simulink library "AeroLib"  (Simulink 6.0)
settings: Solver=ode45  SolverMode=SingleTasking  StartTime=0.0  StopTime=10.0  RelTol=1e-3
undefined symbols (not defined in the file): Aero, Ap, Atm, Control, Controls, Eng, Flight_cg, Flight_DamperON, Flight_delta_isa, Flight_DeltaSpiral, Flight_InertiaSelect, Flight_ixx, Flight_ixz, Flight_iyy, Flight_izz, Flight_latitude, Flight_LoiterLenght, Flight_LoiterMode, Flight_LoiterRadius, Flight_longitude, Flight_MaxTargetPoints, Flight_SensorsON, Flight_TimeStep, Flight_TowerWind_X, Flight_TowerWind_Y, Flight_TowerWind_Z, Flight_TowerWindON, Flight_Trimming, Flight_TurbON, Flight_weight, Flight_WindGustON, Flight_WindShearON, Flight_ycg, Flight_zcg, Geom, Lgear, Mass, PEG_CDwbnp, PEG_CLht, PEG_CLht_elev, PEG_CLwbnp, PEG_CMht, PEG_CMwbnp, PEG_CNbeta, PEG_CNr, PEG_CNrud, PEG_CRail, PEG_CRbeta, PEG_CRp, PEG_CRrud, PEG_CYbeta, PEG_CYrud, pow, Sensors
libraries: AeroLib x133, simulink3 x49, simulink x37, aerospace x11
(part 6 of 7)

== system AeroLib/AtmosphericData/FAA_Std_Gust/Turbulence U/Filter_U2 ==
  Noise : Inport  Port=1  LatchInput=off
  Freq : Inport  Port=2  LatchInput=off
  From_Reset : Inport  Port=3  LatchInput=off
  Constant : Constant  Value=0
  Stateless_Integrator : AeroLib/AMS_StatelessFilters/Stateless_Integrator
  Sum : Sum  Inputs=|+-  SaturateOnIntegerOverflow=on  InputSameDT=on
  err_freq : Product  SaturateOnIntegerOverflow=on  InputSameDT=on
  FiltNoise : Outport
  wires:
  From_Reset/1 -> Stateless_Integrator/1
  Constant/1 -> Stateless_Integrator/2
  err_freq/1 -> Stateless_Integrator/3
  Freq/1 -> err_freq/1
  Sum/1 -> err_freq/2  "err"
  Noise/1 -> Sum/1  "noise_u"
  Stateless_Integrator/1 -> FiltNoise/1, Sum/2

== system AeroLib/AtmosphericData/FAA_Std_Gust/Turbulence V/Filter_V1 ==
  Noise : Inport  Port=1  LatchInput=off
  Freq : Inport  Port=2  LatchInput=off
  From_Reset : Inport  Port=3  LatchInput=off
  Constant : Constant  Value=0
  Stateless_Integrator : AeroLib/AMS_StatelessFilters/Stateless_Integrator
  Sum : Sum  Inputs=|+-  SaturateOnIntegerOverflow=on  InputSameDT=on
  err_freq : Product  SaturateOnIntegerOverflow=on  InputSameDT=on
  FiltNoise : Outport
  wires:
  Stateless_Integrator/1 -> Sum/2, FiltNoise/1
  Noise/1 -> Sum/1  "noise_u"
  Sum/1 -> err_freq/2  "err"
  Freq/1 -> err_freq/1
  err_freq/1 -> Stateless_Integrator/3
  Constant/1 -> Stateless_Integrator/2
  From_Reset/1 -> Stateless_Integrator/1

== system AeroLib/AtmosphericData/FAA_Std_Gust/Turbulence V/Filter_V2 ==
  Noise : Inport  Port=1  LatchInput=off
  Freq : Inport  Port=2  LatchInput=off
  From_Reset : Inport  Port=3  LatchInput=off
  Constant : Constant  Value=0
  Stateless_Integrator : AeroLib/AMS_StatelessFilters/Stateless_Integrator
  Sum : Sum  Inputs=|+-  SaturateOnIntegerOverflow=on  InputSameDT=on
  err_freq : Product  SaturateOnIntegerOverflow=on  InputSameDT=on
  FiltNoise : Outport
  wires:
  From_Reset/1 -> Stateless_Integrator/1
  Constant/1 -> Stateless_Integrator/2
  err_freq/1 -> Stateless_Integrator/3
  Freq/1 -> err_freq/1
  Sum/1 -> err_freq/2  "err"
  Noise/1 -> Sum/1  "noise_u"
  Stateless_Integrator/1 -> FiltNoise/1, Sum/2

== system AeroLib/AtmosphericData/FAA_Std_Gust/Turbulence V/Filter_V3 ==
  Noise : Inport  Port=1  LatchInput=off
  Freq : Inport  Port=2  LatchInput=off
  From_Reset : Inport  Port=3  LatchInput=off
  Constant : Constant  Value=0
  Stateless_Integrator : AeroLib/AMS_StatelessFilters/Stateless_Integrator
  Sum : Sum  Inputs=|+-  SaturateOnIntegerOverflow=on  InputSameDT=on
  err_freq : Product  SaturateOnIntegerOverflow=on  InputSameDT=on
  FiltNoise : Outport
  wires:
  Stateless_Integrator/1 -> Sum/2, FiltNoise/1
  Noise/1 -> Sum/1  "noise_u"
  Sum/1 -> err_freq/2  "err"
  Freq/1 -> err_freq/1
  err_freq/1 -> Stateless_Integrator/3
  Constant/1 -> Stateless_Integrator/2
  From_Reset/1 -> Stateless_Integrator/1

== system AeroLib/AtmosphericData/FAA_Std_Gust/Turbulence W/Filter_W1 ==
  Noise : Inport  Port=1  LatchInput=off
  Freq : Inport  Port=2  LatchInput=off
  From_Reset : Inport  Port=3  LatchInput=off
  Constant : Constant  Value=0
  Stateless_Integrator : AeroLib/AMS_StatelessFilters/Stateless_Integrator
  Sum : Sum  Inputs=|+-  SaturateOnIntegerOverflow=on  InputSameDT=on
  err_freq : Product  SaturateOnIntegerOverflow=on  InputSameDT=on
  FiltNoise : Outport
  wires:
  Stateless_Integrator/1 -> Sum/2, FiltNoise/1
  Noise/1 -> Sum/1  "noise_u"
  Sum/1 -> err_freq/2  "err"
  Freq/1 -> err_freq/1
  err_freq/1 -> Stateless_Integrator/3
  Constant/1 -> Stateless_Integrator/2
  From_Reset/1 -> Stateless_Integrator/1

== system AeroLib/AtmosphericData/FAA_Std_Gust/Turbulence W/Filter_W2 ==
  Noise : Inport  Port=1  LatchInput=off
  Freq : Inport  Port=2  LatchInput=off
  From_Reset : Inport  Port=3  LatchInput=off
  Constant : Constant  Value=0
  Stateless_Integrator : AeroLib/AMS_StatelessFilters/Stateless_Integrator
  Sum : Sum  Inputs=|+-  SaturateOnIntegerOverflow=on  InputSameDT=on
  err_freq : Product  SaturateOnIntegerOverflow=on  InputSameDT=on
  FiltNoise : Outport
  wires:
  From_Reset/1 -> Stateless_Integrator/1
  Constant/1 -> Stateless_Integrator/2
  err_freq/1 -> Stateless_Integrator/3
  Freq/1 -> err_freq/1
  Sum/1 -> err_freq/2  "err"
  Noise/1 -> Sum/1  "noise_u"
  Stateless_Integrator/1 -> FiltNoise/1, Sum/2

== system AeroLib/AtmosphericData/FAA_Std_Gust/Turbulence W/Filter_W3 ==
  Noise : Inport  Port=1  LatchInput=off
  Freq : Inport  Port=2  LatchInput=off
  From_Reset : Inport  Port=3  LatchInput=off
  Constant : Constant  Value=0
  Stateless_Integrator : AeroLib/AMS_StatelessFilters/Stateless_Integrator
  Sum : Sum  Inputs=|+-  SaturateOnIntegerOverflow=on  InputSameDT=on
  err_freq : Product  SaturateOnIntegerOverflow=on  InputSameDT=on
  FiltNoise : Outport
  wires:
  Stateless_Integrator/1 -> Sum/2, FiltNoise/1
  Noise/1 -> Sum/1  "noise_u"
  Sum/1 -> err_freq/2  "err"
  Freq/1 -> err_freq/1
  err_freq/1 -> Stateless_Integrator/3
  Constant/1 -> Stateless_Integrator/2
  From_Reset/1 -> Stateless_Integrator/1

== system AeroLib/Autopilot/Autopilot/Dampers/Pitch_Damper ==
  From_Reset : Inport  Port=1  LatchInput=off
  From_INS : Inport  Port=2  LatchInput=off
  Alpha : Inport  Port=3  LatchInput=off
  From_Prop : Inport  Port=4  LatchInput=off
  From_Inputs : Inport  Port=5  LatchInput=off
  Limit_Alpha_and_Speed : Subsystem
  Pitch_damp : Subsystem  mask{Kq=Ap.Alt.damph, Kd=Ap.Alt.dgain}
      mask prompts: Kq "Damphing"; Kd "Derivative"
  Sum : Sum  Inputs=|++  SaturateOnIntegerOverflow=on  InputSameDT=on
  Elev_cmd : Outport
  wires:
  From_Reset/1 -> Limit_Alpha_and_Speed/2(Reset)
  From_INS/1 -> Limit_Alpha_and_Speed/1(TAS), Pitch_damp/1(From_INS)
  Limit_Alpha_and_Speed/1(Elev_minSpeed) -> Sum/2
  Pitch_damp/1(Elev_cmd) -> Sum/1
  Alpha/1 -> Limit_Alpha_and_Speed/4(Alpha)
  From_Prop/1 -> Limit_Alpha_and_Speed/3(From_Prop)
  Sum/1 -> Elev_cmd/1
  From_Inputs/1 -> Limit_Alpha_and_Speed/5(From_Inputs)

== system AeroLib/Autopilot/Autopilot/Dampers/Roll_Damper ==
  From_Sen : Inport  Port=1  LatchInput=off
  From_Reset : Inport  Port=2  LatchInput=off
  Phi Limit : Subsystem
  Roll_damp : Subsystem  mask{Kp=Ap.Track.damph, Kd=Ap.Track.dgain}
      mask prompts: Kp "Damphing"; Kd "Derivative"
  Sum1 : Sum  Inputs=|++  SaturateOnIntegerOverflow=on  InputSameDT=on
  Ail_cmd : Outport
  wires:
  From_Reset/1 -> Roll_damp/2(Reset_In), Phi Limit/1(Reset_In)
  From_Sen/1 -> Phi Limit/2(Phi), Roll_damp/1(From_Sen)
  Roll_damp/1(Ail_cmd) -> Sum1/1
  Sum1/1 -> Ail_cmd/1
  Phi Limit/1(Ail) -> Sum1/2

== system AeroLib/Autopilot/Autopilot/Dampers/Yaw_Damper ==
  Ny : Inport  Port=1  LatchInput=off
  From_Reset : Inport  Port=2  LatchInput=off
  Gain : Gain  Gain=Ap.Ny.gain  SaturateOnIntegerOverflow=on
  PID_Ny : Subsystem  mask(PID(2) Controller){P=Ap.Ny.pgain, I=Ap.Ny.igain, D=Ap.Ny.dgain}
      mask prompts: P "Proportional:"; I "Integral:"; D "Derivative:"
      mask help:
      | Enter Proportional(P), Integral(I), and Derivative(D) and divisor (N) terms.
      | P+I/s+Ds/(1/Ns+1)
      mask Help: This block implements a PID controller where parameters are entered for the Proportional, Integral and Derivative and divisor terms. Unmask this block to see how it works. The derivative term is implemented using an s/(s/N +1)  transfer function block. Making N large can create a "stiff" system.
      mask Display: disp('PID')
  Rud_cmd : Outport
  wires:
  From_Reset/1 -> PID_Ny/2(From_Reset)
  PID_Ny/1(Cmd) -> Rud_cmd/1
  Ny/1 -> Gain/1
  Gain/1 -> PID_Ny/1(Err)

== system AeroLib/Autopilot/Autopilot/Guidance/Loiter_modes ==
  note: Flight_LoiterMode
      | 1 - Spiral or circle
      | 2 - Serpentine
      | 3 - Lazy eight
  Target_N : Inport  Port=1  LatchInput=off
  From_FSC : Inport  Port=2  LatchInput=off
  From_Reset : Inport  Port=3  LatchInput=off
  Constant : Constant  Value=2
  Constant1 : Constant  Value=Flight_LoiterMode
  Demux : Demux  Outputs=2
  Last_point_data : Subsystem
  MinMax : MinMax  Inputs=2  SaturateOnIntegerOverflow=on  InputSameDT=on
  Multiport Switch : MultiPortSwitch  Inputs=2  SaturateOnIntegerOverflow=on  InputSameDT=on
  Mux : Mux  Inputs=2
  Mux1 : Mux  Inputs=2
  Serpentine_Loiter_mode : Subsystem
  Spiral_and_circle_Loiter_mode : Subsystem  TreatAsAtomicUnit=on
  Subsystem : Subsystem
  Track_Err : Outport
  Point_N : Outport  Port=2
  wires:
  Multiport Switch/1 -> Demux/1
  From_Reset/1 -> Spiral_and_circle_Loiter_mode/3(From_Reset), Serpentine_Loiter_mode/5(From_Reset)
  Mux/1 -> Multiport Switch/2
  Mux1/1 -> Multiport Switch/3
  MinMax/1 -> Multiport Switch/1
  Constant1/1 -> MinMax/1
  Constant/1 -> MinMax/2
  Demux/2 -> Point_N/1
  Demux/1 -> Track_Err/1
  Serpentine_Loiter_mode/2(Point_N) -> Mux1/2
  Serpentine_Loiter_mode/1(Track_Err) -> Mux1/1
  Spiral_and_circle_Loiter_mode/2(Point_N) -> Mux/2
  Spiral_and_circle_Loiter_mode/1(Track_Err) -> Mux/1
  Subsystem/1(Enable_com) -> Spiral_and_circle_Loiter_mode/Enable
  Last_point_data/3(LastTrack_rad) -> Spiral_and_circle_Loiter_mode/1(LastTrack), Serpentine_Loiter_mode/4(Track_last)
  Last_point_data/2(LastY_m) -> Serpentine_Loiter_mode/3(Y_last)
  Last_point_data/1(LastX_m) -> Serpentine_Loiter_mode/2(X_last)
  From_FSC/1 -> Serpentine_Loiter_mode/1(From_FSC), Last_point_data/1(From_Sensors), Spiral_and_circle_Loiter_mode/2(From_FSC)
  Target_N/1 -> Last_point_data/2(Target_N), Subsystem/1(Target_N)

== system AeroLib/Autopilot/Autopilot/Guidance/Target_Errors ==
  Y_req : Inport  Port=1  LatchInput=off
  X_Req : Inport  Port=2  LatchInput=off
  Speed_Req : Inport  Port=3  LatchInput=off
  Alt_Req : Inport  Port=4  LatchInput=off
  From_Prop : Inport  Port=5  LatchInput=off
  From_Inputs : Inport  Port=6  LatchInput=off
  From_Sen : Inport  Port=7  LatchInput=off
  AP_RATO : Subsystem
  Bus Selector3 : BusSelector  DialogController=Simulink.DDGSource_Bus  OutputSignals=IRU_RadarAlt_ft
  Constant : Constant  Value=0
  Switch : Switch  Threshold=0.5  SaturateOnIntegerOverflow=on  InputSameDT=on
  Switch1 : Switch  Threshold=0.5  SaturateOnIntegerOverflow=on  InputSameDT=on
  Target_Errors : AeroLib/Autopilot/Target_Errors
  ft--->m1 : Gain  Gain=1.01  SaturateOnIntegerOverflow=on
  Distance : Outport
  Speed_Err : Outport  Port=2
  Alt_Err : Outport  Port=3
  Bearing : Outport  Port=4
  Time_to_Go : Outport  Port=5
  Track_Err : Outport  Port=6
  wires:
  From_Sen/1 -> AP_RATO/1(FromSensor), Bus Selector3/1, Target_Errors/4
  Bus Selector3/1 -> ft--->m1/1  "<IRU_RadarAlt_ft>"
  AP_RATO/1(HoldAlt_ON) -> Switch1/2, Switch/2
  Target_Errors/6 -> Alt_Err/1
  Target_Errors/5 -> Bearing/1
  Target_Errors/4 -> Speed_Err/1
  Speed_Req/1 -> Target_Errors/3
  X_Req/1 -> Target_Errors/2
  Target_Errors/2 -> Time_to_Go/1
  Target_Errors/1 -> Distance/1
  Y_req/1 -> Target_Errors/1
  Target_Errors/3 -> Switch1/1
  From_Prop/1 -> AP_RATO/2(From_Prop)
  Switch/1 -> Target_Errors/5
  Alt_Req/1 -> Switch/1
  ft--->m1/1 -> Switch/3
  From_Inputs/1 -> AP_RATO/3(From_Inputs)
  Switch1/1 -> Track_Err/1
  Constant/1 -> Switch1/3

== system AeroLib/Autopilot/Autopilot/Guidance/Target_Selector ==
  Distance : Inport  Port=1  LatchInput=off
  PointsXY : Inport  Port=2  LatchInput=off
  PointsLatLon : Inport  Port=3  LatchInput=off
  From_Reset : Inport  Port=4  LatchInput=off
  Counter_Point : AeroLib/Autopilot/Counter_Point  MinDist=Ap.Target.MinDist
  Demux : Demux
  Demux1 : Demux  Outputs=2
  Fcn4 : Fcn  Expr=u+1
  Mem1 : Memory  X0=1000000000
  Saturation : Saturate  UpperLimit=Flight_MaxTargetPoints  LowerLimit=0
  Selector : Selector  InputType=Matrix  Elements=[2 ]  RowSrc=External  Rows=5  Columns=-1  InputPortWidth=4
  Selector1 : Selector  InputType=Matrix  Elements=[2 ]  RowSrc=External  Rows=5  Columns=-1  InputPortWidth=4
  Y_target : Outport
  X_target : Outport  Port=2
  V_req : Outport  Port=3
  Z_target : Outport  Port=4
  Point_N : Outport  Port=5
  Lat_target : Outport  Port=6
  Lon_target : Outport  Port=7
  wires:
  Saturation/1 -> Selector/2, Selector1/2
  Distance/1 -> Mem1/1
  Selector/1 -> Demux/1
  Fcn4/1 -> Saturation/1, Point_N/1
  Demux/1 -> X_target/1
  Demux/2 -> Y_target/1
  Demux/3 -> Z_target/1
  Demux/4 -> V_req/1
  PointsXY/1 -> Selector/1
  Counter_Point/1 -> Fcn4/1
  Mem1/1 -> Counter_Point/1
  From_Reset/1 -> Counter_Point/2
  Selector1/1 -> Demux1/1
  PointsLatLon/1 -> Selector1/1
  Demux1/1 -> Lat_target/1
  Demux1/2 -> Lon_target/1

== system AeroLib/Autopilot/GeodCoor to XY/Geo2orto/Geod_coor ==
  Lat_Init : Inport  Port=1  LatchInput=off
  Lat_Targ : Inport  Port=2  LatchInput=off
  DeltaLon : Inport  Port=3  LatchInput=off
  Product{,1..5} (6 alike) : Product  SaturateOnIntegerOverflow=on  InputSameDT=on
  Sum : Sum  Inputs=|++  SaturateOnIntegerOverflow=on  InputSameDT=on
  Sum1 : Sum  Inputs=|+-  SaturateOnIntegerOverflow=on  InputSameDT=on
  Trigonometric Function1 : Trigonometry
  Trigonometric Function2 : Trigonometry  Operator=cos
  Trigonometric Function3 : Trigonometry  Operator=cos
  Trigonometric Function4 : Trigonometry
  Trigonometric Function5 : Trigonometry
  Trigonometric Function6 : Trigonometry  Operator=cos
  P : Outport
  U : Outport  Port=2
  Q : Outport  Port=3
  wires:
  Trigonometric Function4/1 -> Product3/1, Product5/1
  Trigonometric Function6/1 -> Product2/2, Product4/2
  Lat_Init/1 -> Trigonometric Function4/1, Trigonometric Function6/1
  Trigonometric Function5/1 -> Product3/2, Product2/1
  Lat_Targ/1 -> Trigonometric Function3/1, Trigonometric Function5/1
  Trigonometric Function3/1 -> Product/1, Product1/1
  Trigonometric Function1/1 -> Product/2
  DeltaLon/1 -> Trigonometric Function1/1, Trigonometric Function2/1
  Trigonometric Function2/1 -> Product1/2
  Product/1 -> P/1
  Product3/1 -> Sum/1
  Product1/1 -> Product4/1, Product5/2
  Product4/1 -> Sum/2
  Sum/1 -> U/1
  Product2/1 -> Sum1/1
  Product5/1 -> Sum1/2
  Sum1/1 -> Q/1

== system AeroLib/EquationsOfMotion/Equations_of_Motion/EQM Six-DOF/EQM Forces ==
  Fext : Inport  Port=1  LatchInput=off
  Weight : Inport  Port=2  LatchInput=off
  Rate : Inport  Port=3  LatchInput=off
  Vb : Inport  Port=4  LatchInput=off
  Force_Vb_w : aerospace/Axes Transformations/3x3 cross product
  Gravity : Constant  Value=Atm.grav
  Product : Product  Inputs=*/  SaturateOnIntegerOverflow=on  InputSameDT=on
  Product1 : Product  Inputs=*/  SaturateOnIntegerOverflow=on  InputSameDT=on
  sum : Sum  SaturateOnIntegerOverflow=on  InputSameDT=on
  Accel : Outport
  wires:
  sum/1 -> Accel/1
  Product/1 -> sum/1
  Force_Vb_w/1 -> sum/2
  Fext/1 -> Product/1
  Vb/1 -> Force_Vb_w/1
  Rate/1 -> Force_Vb_w/2
  Weight/1 -> Product1/1
  Gravity/1 -> Product1/2
  Product1/1 -> Product/2

== system AeroLib/EquationsOfMotion/Equations_of_Motion/EQM Six-DOF/EQM Moments ==
  Moments : Inport  Port=1  LatchInput=off
  Inertia : Inport  Port=2  LatchInput=off
  Rates : Inport  Port=3  LatchInput=off
  Moment_Rates_Inertia : aerospace/Axes Transformations/3x3 cross product
  Product : Product  Inputs=/*  Multiplication=Matrix(*)  SaturateOnIntegerOverflow=on  InputSameDT=on
  matr_mult : Product  Multiplication=Matrix(*)  SaturateOnIntegerOverflow=on  InputSameDT=on
  sum1 : Sum  Inputs=+-  SaturateOnIntegerOverflow=on  InputSameDT=on
  pdot qdot rdot : Outport
  wires:
  Product/1 -> pdot qdot rdot/1
  Moment_Rates_Inertia/1 -> sum1/2
  matr_mult/1 -> Moment_Rates_Inertia/2
  Moments/1 -> sum1/1
  Rates/1 -> Moment_Rates_Inertia/1, matr_mult/2
  Inertia/1 -> matr_mult/1, Product/1
  sum1/1 -> Product/2

== system AeroLib/EquationsOfMotion/Equations_of_Motion/EQM Six-DOF/Geodetic_Frame_EQM ==
  note: LongitudeDot
      |
      |
      | LatitudeDot
  note: XYZ - Earth axis system
      |
      | X - pointing North
      | Y - pointing East
      | Z - pointing Down towards the center of the Earth
  VN : Inport  Port=1  LatchInput=off
  VE : Inport  Port=2  LatchInput=off
  Alt_m : Inport  Port=3  LatchInput=off
  Reset : Inport  Port=4  LatchInput=off
  Constant : Constant  Value=0
  Constant1 : Constant  Value=Flight_latitude
  Constant23 : Constant  Value=Flight_longitude
  Deg-->Rad : Gain  Gain=pi/180  SaturateOnIntegerOverflow=on
  Demux : Demux  Outputs=2
  Fcn5 : Fcn  Expr=u(2)*sin(u(1))
  LatitudeDot : Product  Inputs=/*  SaturateOnIntegerOverflow=on  InputSameDT=on
  LongitudeDot : Product  Inputs=*//  SaturateOnIntegerOverflow=on  InputSameDT=on
  Longitude_Bound : Subsystem
  Mux{,1..2,4} (4 alike) : Mux  Inputs=2
  Stateless_Integrator : AeroLib/AMS_StatelessFilters/Stateless_Integrator
  Stateless_Integrator1 : AeroLib/AMS_StatelessFilters/Stateless_Integrator
  Trigonometric Function : Trigonometry  Operator=cos
  WGS 84 : Subsystem
  Zero-->Eps : Subsystem
  latitude_Bound : Lookup  DialogController=Simulink.DDGSource  InputValues=[-2*pi -3*pi/2 -pi -pi/2 0 pi/2 pi 3*pi/2 2*pi]  OutputValues=[0 pi/2 0 -pi/2 0 pi/2 0 -pi/2 0]  SaturateOnIntegerOverflow=on
  rad-->deg : Gain  Gain=180/pi  SaturateOnIntegerOverflow=on
  Wander angle_rad : Outport
  Latitude_deg : Outport  Port=2
  Longitude_deg : Outport  Port=3
  GeodHeight_m : Outport  Port=4
  wires:
  Alt_m/1 -> WGS 84/2(Altitude_m)
  VN/1 -> LatitudeDot/2
  WGS 84/3(RadOfCurv_mer_m) -> LatitudeDot/1
  Longitude_Bound/2(Lat_deg) -> Latitude_deg/1
  Mux1/1 -> rad-->deg/1
  LongitudeDot/1 -> Mux4/2, Mux/1
  Mux/1 -> Stateless_Integrator1/3
  LatitudeDot/1 -> Mux/2
  Stateless_Integrator1/1 -> Demux/1
  Trigonometric Function/1 -> Zero-->Eps/1(In1)
  WGS 84/2(GeogHight_m) -> GeodHeight_m/1
  Zero-->Eps/1(Out1) -> LongitudeDot/2
  WGS 84/1(RadOfCurv_ver_m) -> LongitudeDot/3
  Demux/2 -> latitude_Bound/1  "Lat"
  VE/1 -> LongitudeDot/1
  rad-->deg/1 -> Longitude_Bound/1(Lat Lon)
  Demux/1 -> Mux1/2  "Longitude"
  Mux4/1 -> Fcn5/1
  Stateless_Integrator/1 -> Wander angle_rad/1
  latitude_Bound/1 -> Mux1/1, Mux4/1, Trigonometric Function/1, WGS 84/1(Latitude_rad)  "Latitude"
  Longitude_Bound/1(Lon_deg) -> Longitude_deg/1
  Fcn5/1 -> Stateless_Integrator/3
  Reset/1 -> Stateless_Integrator/1, Stateless_Integrator1/1
  Constant/1 -> Stateless_Integrator/2
  Constant23/1 -> Mux2/1
  Constant1/1 -> Mux2/2
  Mux2/1 -> Deg-->Rad/1
  Deg-->Rad/1 -> Stateless_Integrator1/2

== system AeroLib/EquationsOfMotion/Equations_of_Motion/EQM Six-DOF/Quaternion_Euler ==
  P Q R : Inport  Port=1  LatchInput=off
  From_Reset : Inport  Port=2  LatchInput=off
  Clock : Clock
      settings: Decimation=10
  Constant : Constant  Value=Flight_Trimming
  EUL2QUA : AeroLib/CoordinateSystems/EUL2QUA
  Euler : Subsystem  TreatAsAtomicUnit=on
  Fcn : Fcn  Expr=u <= 0
  Gain : Gain  Gain=180/pi  SaturateOnIntegerOverflow=on
  Logical Operator : Logic  Orientation=left  Operator=NOT
  Quaternion_Comp : Subsystem  TreatAsAtomicUnit=on
  Stateless_HighPass : AeroLib/AMS_StatelessFilters/Stateless_HighPass
  Switch : Switch  Threshold=0.5  SaturateOnIntegerOverflow=on  InputSameDT=on
  Switch1 : Switch  Threshold=0.5  SaturateOnIntegerOverflow=on  InputSameDT=on
  Tau : Constant  Value=0.1
  or : Logic  Operator=OR
  Euler_rad : Outport
  Quaternion : Outport  Port=2  InitialOutput=0
  Euler_deg : Outport  Port=3
  EulerDot_degps : Outport  Port=4
  wires:
  Tau/1 -> Stateless_HighPass/3
  From_Reset/1 -> Stateless_HighPass/1
  Stateless_HighPass/1 -> EulerDot_degps/1
  Switch/1 -> Gain/1, Euler_rad/1
  Gain/1 -> Stateless_HighPass/2, Euler_deg/1
  P Q R/1 -> Quaternion_Comp/2(P Q R), Euler/1(P Q R)
  Quaternion_Comp/1(Euler  angles) -> Switch/3
  Quaternion_Comp/2(Quaternion) -> Switch1/3
  or/1 -> Switch/2, Switch1/2, Logical Operator/1, Euler/Enable
  Euler/1(Euler_Trim) -> Switch/1, EUL2QUA/1
  Clock/1 -> Fcn/1
  Constant/1 -> or/1  "DT"
  Fcn/1 -> or/2
  EUL2QUA/1 -> Quaternion_Comp/1(Flight_q), Switch1/1
  Switch1/1 -> Quaternion/1
  Logical Operator/1 -> Quaternion_Comp/Enable

== system AeroLib/EquationsOfMotion/Equations_of_Motion/EQM Six-DOF/Velocity Computation ==
  Wander angle_rad : Inport  Port=1  LatchInput=off
  Vb : Inport  Port=2  LatchInput=off
  phi theta psi : Inport  Port=3  LatchInput=off
  BOA2LEF : AeroLib/CoordinateSystems/BOA2LEF
  Constant : Constant  Value=0
  Constant1 : Constant  Value=0
  EUL2DCM : AeroLib/CoordinateSystems/EUL2DCM
  Mux : Mux  Inputs=3
  Sum : Sum  Inputs=|++  SaturateOnIntegerOverflow=on  InputSameDT=on
  Vel_NED : Outport
  wires:
  BOA2LEF/1 -> Vel_NED/1
  Vb/1 -> BOA2LEF/1
  EUL2DCM/1 -> BOA2LEF/2
  Mux/1 -> Sum/2
  Wander angle_rad/1 -> Mux/3
  Constant1/1 -> Mux/2
  Constant/1 -> Mux/1
  phi theta psi/1 -> Sum/1
  Sum/1 -> EUL2DCM/1

== system AeroLib/EquationsOfMotion/Equations_of_Motion/EQM_Outputs/Inertilal Positions ==
  AG_b : Inport  Port=1  LatchInput=off
  DCM : Inport  Port=2  LatchInput=off
  Ve : Inport  Port=3  LatchInput=off
  Xe : Inport  Port=4  LatchInput=off
  PsiRad : Inport  Port=5  LatchInput=off
  Accelerations : Subsystem
  FlightPathVel : Subsystem
  HeadingAcc : Subsystem
  Positions : Subsystem
  TrackAcc : Subsystem
  Velocities : Subsystem
  Xdist_m : Outport  InitialOutput=0
  Ydist_m : Outport  Port=2  InitialOutput=0
  Hagl_m : Outport  Port=3  InitialOutput=0
  Hagl_ft : Outport  Port=4  InitialOutput=0
  Hdot_mps : Outport  Port=5  InitialOutput=0
  Hdot_ftpmin : Outport  Port=6  InitialOutput=0
  GroundSpeed_kt : Outport  Port=7  InitialOutput=0
  Gamma_deg : Outport  Port=8  InitialOutput=0
  Track_deg : Outport  Port=9  InitialOutput=0
  AlongTrackAcc_g : Outport  Port=10  InitialOutput=0
  CrossTrackAcc_g : Outport  Port=11  InitialOutput=0
  CrossTrackVel_mps : Outport  Port=12  InitialOutput=0
  AlongPathAcc_g : Outport  Port=13  InitialOutput=0
  VertAcc_g : Outport  Port=14  InitialOutput=0
  AlongHeadAcc_g : Outport  Port=15  InitialOutput=0
  CrossHeadAcc_g : Outport  Port=16  InitialOutput=0
  wires:
  Velocities/9(Gamma_rad) -> FlightPathVel/2(Ang_rad)
  Velocities/8(Ydot_mps) -> TrackAcc/3(Ydot)
  Velocities/7(Xdot_mps) -> TrackAcc/2(Xdot)
  Velocities/6(Track_rad) -> TrackAcc/1(Ang_rad)
  Ve/1 -> Velocities/1(Vi)  "Ve"
  Velocities/5(Hdot_ftpmin) -> Hdot_ftpmin/1
  Velocities/4(Track_deg) -> Track_deg/1
  Velocities/3(Gamma_deg) -> Gamma_deg/1
  Velocities/2(GroundSpeed_kt) -> GroundSpeed_kt/1
  Velocities/1(Hdot_mps) -> Hdot_mps/1
  AG_b/1 -> Accelerations/2(AG_b)
  DCM/1 -> Accelerations/1(DCM)
  Positions/4(Hagl_ft) -> Hagl_ft/1
  Positions/3(Hagl_m) -> Hagl_m/1
  Xe/1 -> Positions/1(Xe)
  Positions/2(Ydist) -> Ydist_m/1
  Positions/1(Xdist) -> Xdist_m/1
  TrackAcc/3(CrossTrackVel) -> CrossTrackVel_mps/1
  HeadingAcc/2(Cross) -> CrossHeadAcc_g/1
  HeadingAcc/1(Along) -> AlongHeadAcc_g/1
  PsiRad/1 -> HeadingAcc/3(Ang_rad)
  Accelerations/3(Zacc) -> FlightPathVel/3(Zacc)
  FlightPathVel/2(VertAcc_g) -> VertAcc_g/1
  FlightPathVel/1(AlongPathAcc_g) -> AlongPathAcc_g/1
  TrackAcc/2(CrossAcc) -> CrossTrackAcc_g/1
  TrackAcc/1(AlongAcc) -> AlongTrackAcc_g/1, FlightPathVel/1(AlongTrackAcc)
  Accelerations/1(Xacc) -> TrackAcc/4(Xacc), HeadingAcc/1(Xacc)
  Accelerations/2(Yacc) -> HeadingAcc/2(Yacc), TrackAcc/5(Yacc)

== system AeroLib/GroundReactions/Landing_Gear/GHM Dir_Cos/DCM Ground_to_Inertial ==
  note: Transformation from
      | Euler Angles (phi, theta, psi) to
      | Directional Cosinus Matrix
  phi theta psi : Inport  Port=1  LatchInput=off
  11 : Fcn  Expr=cos(u[3])*cos(u[2])
  12 : Fcn  Expr=cos(u[3])*sin(u[2])*sin(u[1])-sin(u[3])*cos(u[1])
  13 : Fcn  Expr=cos(u[3])*sin(u[2])*cos(u[1])+sin(u[3])*sin(u[1])
  21 : Fcn  Expr=sin(u[3])*cos(u[2])
  22 : Fcn  Expr=sin(u[3])*sin(u[2])*sin(u[1])+cos(u[3])*cos(u[1])
  23 : Fcn  Expr=sin(u[3])*sin(u[2])*cos(u[1])-cos(u[3])*sin(u[1])
  31 : Fcn  Expr=-sin(u[2])
  32 : Fcn  Expr=cos(u[2])*sin(u[1])
  33 : Fcn  Expr=cos(u[2])*cos(u[1])
  Mux2 : Mux  Inputs=9
  Reshape : simulink3/Signals & Systems/Reshape  OutputDimensionality=Customize  OutputDimensions=[3,3]
  DCM : Outport  InitialOutput=0
  wires:
  33/1 -> Mux2/9
  11/1 -> Mux2/1
  phi theta psi/1 -> 11/1, 12/1, 13/1, 22/1, 23/1, 31/1, 33/1, 32/1, 21/1
  22/1 -> Mux2/5
  12/1 -> Mux2/2
  13/1 -> Mux2/3
  21/1 -> Mux2/4
  23/1 -> Mux2/6
  31/1 -> Mux2/7
  32/1 -> Mux2/8
  Mux2/1 -> Reshape/1
  Reshape/1 -> DCM/1

== system AeroLib/GroundReactions/Landing_Gear/GHM Dir_Cos/INIT_LGEAR ==
  Constant : Constant  Value=Lgear(1).Tire.RposLmg
  Constant1 : Constant  Value=Lgear(2).Tire.RposNg
  Constant2 : Constant  Value=Lgear(1).Tire.RposRmg
  Constant4 : Constant  Orientation=left  Value=Flight_cg
  Constant5 : Constant  Value=Flight_ycg
  Constant6 : Constant  Value=Flight_zcg
  Mux1 : Mux  Inputs=3
  Sum : Sum  Inputs=+-  SaturateOnIntegerOverflow=on  InputSameDT=on
  Sum1 : Sum  Inputs=+-  SaturateOnIntegerOverflow=on  InputSameDT=on
  Sum2 : Sum  Inputs=+-  SaturateOnIntegerOverflow=on  InputSameDT=on
  xcg2ac : Fcn  Expr=(u-0.25)*Geom.Wing.cref+Geom.Wing.xwac
  TireRposLmg : Outport
  TireRposNg : Outport  Port=2
  TireRposRmg : Outport  Port=3
  wires:
  Mux1/1 -> Sum/1, Sum2/1, Sum1/1  "Rcg"
  Sum/1 -> TireRposLmg/1
  Sum2/1 -> TireRposNg/1
  Sum1/1 -> TireRposRmg/1
  Constant/1 -> Sum/2
  Constant1/1 -> Sum2/2
  Constant2/1 -> Sum1/2
  Constant4/1 -> xcg2ac/1  "xcg"
  xcg2ac/1 -> Mux1/1
  Constant5/1 -> Mux1/2
  Constant6/1 -> Mux1/3

== system AeroLib/GroundReactions/Landing_Gear/GHM Ground_Reactions/Moments ==
  FgearLmg : Inport  Port=1  LatchInput=off
  FgearNg : Inport  Port=2  LatchInput=off
  FgearRmg : Inport  Port=3  LatchInput=off
  Rlmg : Inport  Port=4  LatchInput=off
  Rng : Inport  Port=5  LatchInput=off
  Rrmg : Inport  Port=6  LatchInput=off
  LMG_Moment : aerospace/Axes Transformations/3x3 cross product
  NG_Moment : aerospace/Axes Transformations/3x3 cross product
  RMG_Moment : aerospace/Axes Transformations/3x3 cross product
  Sum1 : Sum  Inputs=+++  SaturateOnIntegerOverflow=on  InputSameDT=on
  Mgear : Outport
  wires:
  LMG_Moment/1 -> Sum1/1  "Mgear_LMG"
  NG_Moment/1 -> Sum1/2  "Mgear_NG"
  RMG_Moment/1 -> Sum1/3  "Mgear_RMG"
  Sum1/1 -> Mgear/1
  Rrmg/1 -> RMG_Moment/1
  FgearRmg/1 -> RMG_Moment/2
  FgearNg/1 -> NG_Moment/2
  FgearLmg/1 -> LMG_Moment/2
  Rlmg/1 -> LMG_Moment/1
  Rng/1 -> NG_Moment/1

== system AeroLib/GroundReactions/Landing_Gear/GHM Ground_Reactions/Reactions1 ==
  MUeLmg : Inport  Port=1  LatchInput=off
  MUsLmg : Inport  Port=2  LatchInput=off
  FstrLmg : Inport  Port=3  LatchInput=off
  MUeNg : Inport  Port=4  LatchInput=off
  MUsNg : Inport  Port=5  LatchInput=off
  FstrNg : Inport  Port=6  LatchInput=off
  MUeRmg : Inport  Port=7  LatchInput=off
  MUsRmg : Inport  Port=8  LatchInput=off
  FstrRmg : Inport  Port=9  LatchInput=off
  EulerRad : Inport  Port=10  LatchInput=off
  NoseWheelAng : Inport  Port=11  LatchInput=off
  Gain1 : Gain  Gain=-1  SaturateOnIntegerOverflow=on
  Gain2 : Gain  Gain=-1  SaturateOnIntegerOverflow=on
  Inertial2Body : Subsystem
  Mux1 : Mux  Inputs=3
  Mux2 : Mux  Inputs=3
  NoseGearForces : Subsystem
  Product{1..7} (7 alike) : Product  SaturateOnIntegerOverflow=on  InputSameDT=on
  cosThecosPhi : Fcn  Expr=cos(u(1))*cos(u(2))
  Fgear : Outport
  FgearLMG : Outport  Port=2
  FgearNG : Outport  Port=3
  FgearRMG : Outport  Port=4
  wires:
  Inertial2Body/1(Fg_B) -> Fgear/1
  Inertial2Body/4(FgRMG_B) -> FgearRMG/1
  Inertial2Body/2(FgLMG_B) -> FgearLMG/1
  Inertial2Body/3(FgNG_B) -> FgearNG/1
  NoseWheelAng/1 -> NoseGearForces/4(NoseWheelAng)
  cosThecosPhi/1 -> Product6/1, Product7/2, Product5/1
  FstrNg/1 -> Product6/2
  FstrLmg/1 -> Product7/1
  FstrRmg/1 -> Product5/2
  Product7/1 -> Product3/2, Product1/2, Mux1/3
  Product6/1 -> NoseGearForces/3(FstrNg)
  Product5/1 -> Product4/2, Product2/2, Mux2/3
  EulerRad/1 -> Inertial2Body/4(EulerRad), cosThecosPhi/1
  Gain1/1 -> Inertial2Body/3(FgRMG_I)  "FgearRMG_I"
  MUsRmg/1 -> Product4/1
  MUeRmg/1 -> Product2/1
  Mux2/1 -> Gain1/1
  Product4/1 -> Mux2/2
  Product2/1 -> Mux2/1  "RmgXi"
  MUeLmg/1 -> Product1/1
  MUsLmg/1 -> Product3/1
  Gain2/1 -> Inertial2Body/1(FgLMG_I)  "FgearLMG_I"
  Mux1/1 -> Gain2/1
  Product3/1 -> Mux1/2
  Product1/1 -> Mux1/1  "LmgXi"
  MUeNg/1 -> NoseGearForces/1(MUeNg)
  MUsNg/1 -> NoseGearForces/2(MUsNg)
  NoseGearForces/1(FgearNG) -> Inertial2Body/2(FgNG_I)  "FgearNG_I"

== system AeroLib/GroundReactions/Landing_Gear/Left Main Gear Dynamics/Ground_Tire Contact ==
  DCbg : Inport  Port=1  LatchInput=off
  VelB : Inport  Port=2  LatchInput=off
  RatesB : Inport  Port=3  LatchInput=off
  Sdot : Inport  Port=4  LatchInput=off
  S : Inport  Port=5  LatchInput=off
  TireComp : Inport  Port=6  LatchInput=off
  Conf_Tire_RposLmg : Inport  Port=7  LatchInput=off
  " (97)1" : Sum  Inputs=|+-  SaturateOnIntegerOverflow=on  InputSameDT=on
  " (97)2" : Sum  Inputs=|++  SaturateOnIntegerOverflow=on  InputSameDT=on
  " (98) Mux_3" : Mux  Inputs=3
  3x3 cross product : aerospace/Axes Transformations/3x3 cross product
  Fcn : Fcn  Expr=u(1)
  Fcn1 : Fcn  Expr=u(2)
  Fcn2 : Fcn  Expr=u(3)-u(4)-u(5)
  Product1 : Product  Multiplication=Matrix(*)  SaturateOnIntegerOverflow=on  InputSameDT=on
  Tire Position Body_Axis (95) Mux_1 : Mux  Inputs=3
  Tire Transl_Speed Body_Axis (96) Demux1 : Demux  Outputs=3
  Tire Transl_Speed Body_Axis (96) Mux_2 : Mux  Inputs=3
  Rtb : Outport
  Vtg : Outport  Port=2
  wires:
  Tire Transl_Speed Body_Axis (96) Demux1/1 -> Tire Transl_Speed Body_Axis (96) Mux_2/1
  Tire Transl_Speed Body_Axis (96) Demux1/2 -> Tire Transl_Speed Body_Axis (96) Mux_2/2
  Tire Transl_Speed Body_Axis (96) Demux1/3 -> " (97)1"/1
  Sdot/1 -> " (97)1"/2  "Sdot"
  " (97)1"/1 -> Tire Transl_Speed Body_Axis (96) Mux_2/3
  Tire Transl_Speed Body_Axis (96) Mux_2/1 -> " (97)2"/1  "Vtbtrans"
  TireComp/1 -> Tire Position Body_Axis (95) Mux_1/3
  S/1 -> Tire Position Body_Axis (95) Mux_1/2
  Tire Position Body_Axis (95) Mux_1/1 -> Fcn/1, Fcn1/1, Fcn2/1
  Fcn/1 -> " (98) Mux_3"/1
  Fcn1/1 -> " (98) Mux_3"/2
  Fcn2/1 -> " (98) Mux_3"/3
  " (98) Mux_3"/1 -> Rtb/1, 3x3 cross product/1  "Rtb"
  3x3 cross product/1 -> " (97)2"/2
  " (97)2"/1 -> Product1/2  "Vtb"
  DCbg/1 -> Product1/1
  Product1/1 -> Vtg/1
  Conf_Tire_RposLmg/1 -> Tire Position Body_Axis (95) Mux_1/1
  VelB/1 -> Tire Transl_Speed Body_Axis (96) Demux1/1
  RatesB/1 -> 3x3 cross product/2

== system AeroLib/GroundReactions/Landing_Gear/Left Main Gear Dynamics/Ground_Tire Friction ==
  TireForce : Inport  Port=1  PortDimensions=1  LatchInput=off
  Vtg : Inport  Port=2  PortDimensions=3  LatchInput=off
  Brake : Inport  Port=3  PortDimensions=1  LatchInput=off
  Demux : Demux  Outputs=3
  Friction Coeff : Subsystem
  Terminator : Terminator
  MUside : Outport
  MUeff : Outport  Port=2
  wires:
  Friction Coeff/1(MUside) -> MUside/1
  Friction Coeff/2(MUeff) -> MUeff/1
  Brake/1 -> Friction Coeff/1(Brake)
  Vtg/1 -> Demux/1
  TireForce/1 -> Friction Coeff/4(TireForce)
  Demux/1 -> Friction Coeff/2(Ug)  "Ug"
  Demux/2 -> Friction Coeff/3(Vg)  "Vg"
  Demux/3 -> Terminator/1  "Wg"

== system AeroLib/GroundReactions/Landing_Gear/Left Main Gear Dynamics/LGEAR Accelerations ==
  Hagl : Inport  Orientation=left  Port=1  LatchInput=off
  Sdot : Inport  Orientation=left  Port=2  PortDimensions=1  LatchInput=off
  S : Inport  Orientation=left  Port=3  PortDimensions=1  LatchInput=off
  " (36)" : Sum  Orientation=left  Inputs=+-  SaturateOnIntegerOverflow=on  InputSameDT=on
  " (96)" : Gain  Orientation=left  Gain=Damping  SaturateOnIntegerOverflow=on
  " (96)1" : Gain  Orientation=left  Gain=Tire_Stiffness  SaturateOnIntegerOverflow=on
  " (96)2" : Gain  Orientation=left  Gain=CFriction  SaturateOnIntegerOverflow=on
  " (99)" : Sum  Orientation=left  Inputs=+-  SaturateOnIntegerOverflow=on  InputSameDT=on
  " (99)1" : Sum  Orientation=left  Inputs=|+-  SaturateOnIntegerOverflow=on  InputSameDT=on
  " (99)2" : Sum  Orientation=left  SaturateOnIntegerOverflow=on  InputSameDT=on
  Abs : Abs  Orientation=left  SaturateOnIntegerOverflow=on
  Fcn : Fcn  Orientation=left  Expr=u/Mass/AccFactor
  Product : Product  Orientation=left  SaturateOnIntegerOverflow=on  InputSameDT=on
  Saturation : Saturate  Orientation=left  UpperLimit=TireMaxComp  LowerLimit=0
  Stiffness vs Deflection : Lookup  Orientation=left  DialogController=Simulink.DDGSource  InputValues=Strut_Deflection  OutputValues=Strut_Stiffness  SaturateOnIntegerOverflow=on
  TireForce : Outport  Orientation=left
  S2dot : Outport  Orientation=left  Port=2
  TireComp : Outport  Orientation=left  Port=3
  wires:
  " (36)"/1 -> Fcn/1  "Strut_force"
  " (99)"/1 -> " (36)"/1  "Delta_force"
  Stiffness vs Deflection/1 -> " (99)"/2  "Stiffness"
  Fcn/1 -> S2dot/1
  S/1 -> " (99)1"/2, Stiffness vs Deflection/1
  " (96)1"/1 -> " (99)"/1, TireForce/1  "TireForce"
  " (99)1"/1 -> Saturation/1  "TireComp"
  Hagl/1 -> " (99)1"/1
  Saturation/1 -> " (96)1"/1, TireComp/1
  Product/1 -> " (96)"/1
  Abs/1 -> Product/2
  Sdot/1 -> Product/1, Abs/1, " (96)2"/1
  " (96)"/1 -> " (99)2"/1  "Damping"
  " (96)2"/1 -> " (99)2"/2
  " (99)2"/1 -> " (36)"/2

== system AeroLib/GroundReactions/Landing_Gear/Left Main Gear Dynamics/LGEAR States ==
  S2dot : Inport  Port=1  PortDimensions=1  SampleTime=[Flight_TimeStep,0]  LatchInput=off
  LMG_S : Integrator  LimitOutput=on  UpperSaturationLimit=Strut_Limit  LowerSaturationLimit=0
  LMG_Sdot : Integrator  UpperSaturationLimit=100  LowerSaturationLimit=-100
  Sdot : Outport
  S : Outport  Port=2
  wires:
  LMG_S/1 -> S/1  "S"
  S2dot/1 -> LMG_Sdot/1
  LMG_Sdot/1 -> LMG_S/1, Sdot/1  "Sdot"

== system AeroLib/GroundReactions/Landing_Gear/Nose Gear Dynamics/Ground_Tire Contact ==
  DCbg : Inport  Port=1  LatchInput=off
  VelB : Inport  Port=2  LatchInput=off
  RatesB : Inport  Port=3  LatchInput=off
  Sdot : Inport  Port=4  LatchInput=off
  S : Inport  Port=5  LatchInput=off
  TireComp : Inport  Port=6  LatchInput=off
  Conf_Tire_RposNg : Inport  Port=7  LatchInput=off
  " (97)1" : Sum  Inputs=|+-  SaturateOnIntegerOverflow=on  InputSameDT=on
  " (97)2" : Sum  Inputs=|++  SaturateOnIntegerOverflow=on  InputSameDT=on
  " (98) Mux_3" : Mux  Inputs=3
  3x3 cross product : aerospace/Axes Transformations/3x3 cross product
  Fcn : Fcn  Expr=u(1)
  Fcn1 : Fcn  Expr=u(2)
  Fcn2 : Fcn  Expr=u(3)-u(4)-u(5)
  Product1 : Product  Multiplication=Matrix(*)  SaturateOnIntegerOverflow=on  InputSameDT=on
  Tire Position Body_Axis (95) Mux_1 : Mux  Inputs=3
  Tire Transl_Speed Body_Axis (96) Demux1 : Demux  Outputs=3
  Tire Transl_Speed Body_Axis (96) Mux_2 : Mux  Inputs=3
  Rtb : Outport
  Vtg : Outport  Port=2
  wires:
  Tire Transl_Speed Body_Axis (96) Demux1/1 -> Tire Transl_Speed Body_Axis (96) Mux_2/1
  Tire Transl_Speed Body_Axis (96) Demux1/2 -> Tire Transl_Speed Body_Axis (96) Mux_2/2
  Tire Transl_Speed Body_Axis (96) Demux1/3 -> " (97)1"/1
  Sdot/1 -> " (97)1"/2  "Sdot"
  " (97)1"/1 -> Tire Transl_Speed Body_Axis (96) Mux_2/3
  Tire Transl_Speed Body_Axis (96) Mux_2/1 -> " (97)2"/1  "Vtbtrans"
  TireComp/1 -> Tire Position Body_Axis (95) Mux_1/3
  S/1 -> Tire Position Body_Axis (95) Mux_1/2
  Tire Position Body_Axis (95) Mux_1/1 -> Fcn/1, Fcn1/1, Fcn2/1
  Fcn/1 -> " (98) Mux_3"/1
  Fcn1/1 -> " (98) Mux_3"/2
  Fcn2/1 -> " (98) Mux_3"/3
  " (98) Mux_3"/1 -> Rtb/1, 3x3 cross product/1  "Rtb"
  3x3 cross product/1 -> " (97)2"/2
  " (97)2"/1 -> Product1/2  "Vtb"
  DCbg/1 -> Product1/1
  Product1/1 -> Vtg/1
  Conf_Tire_RposNg/1 -> Tire Position Body_Axis (95) Mux_1/1
  VelB/1 -> Tire Transl_Speed Body_Axis (96) Demux1/1
  RatesB/1 -> 3x3 cross product/2

== system AeroLib/GroundReactions/Landing_Gear/Nose Gear Dynamics/Ground_Tire Friction ==
  TireForce : Inport  Port=1  PortDimensions=1  LatchInput=off
  Vtg : Inport  Port=2  PortDimensions=3  LatchInput=off
  Demux : Demux  Outputs=3
  Friction Coeff : Subsystem
  Terminator : Terminator
  MUside : Outport
  MUeff : Outport  Port=2
  wires:
  Demux/3 -> Terminator/1  "Wg"
  Demux/2 -> Friction Coeff/2(Vg)  "Vg"
  Demux/1 -> Friction Coeff/1(Ug)  "Ug"
  TireForce/1 -> Friction Coeff/3(TireForce)
  Vtg/1 -> Demux/1
  Friction Coeff/2(MUeff) -> MUeff/1
  Friction Coeff/1(MUside) -> MUside/1

== system AeroLib/GroundReactions/Landing_Gear/Nose Gear Dynamics/LGEAR Accelerations ==
  Hagl : Inport  Orientation=left  Port=1  LatchInput=off
  Sdot : Inport  Orientation=left  Port=2  PortDimensions=1  LatchInput=off
  S : Inport  Orientation=left  Port=3  PortDimensions=1  LatchInput=off
  " (36)" : Sum  Orientation=left  Inputs=+-  SaturateOnIntegerOverflow=on  InputSameDT=on
  " (96)" : Gain  Orientation=left  Gain=Damping  SaturateOnIntegerOverflow=on
  " (96)1" : Gain  Orientation=left  Gain=Tire_Stiffness  SaturateOnIntegerOverflow=on
  " (96)2" : Gain  Orientation=left  Gain=CFriction  SaturateOnIntegerOverflow=on
  " (99)" : Sum  Orientation=left  Inputs=+-  SaturateOnIntegerOverflow=on  InputSameDT=on
  " (99)1" : Sum  Orientation=left  Inputs=|+-  SaturateOnIntegerOverflow=on  InputSameDT=on
  " (99)2" : Sum  Orientation=left  SaturateOnIntegerOverflow=on  InputSameDT=on
  Abs : Abs  Orientation=left  SaturateOnIntegerOverflow=on
  Fcn : Fcn  Orientation=left  Expr=u/Mass/AccFactor
  Product : Product  Orientation=left  SaturateOnIntegerOverflow=on  InputSameDT=on
  Saturation : Saturate  Orientation=left  UpperLimit=TireMaxComp  LowerLimit=0
  Stiffness vs Deflection : Lookup  Orientation=left  DialogController=Simulink.DDGSource  InputValues=Strut_Deflection  OutputValues=Strut_Stiffness  SaturateOnIntegerOverflow=on
  TireForce : Outport  Orientation=left
  S2dot : Outport  Orientation=left  Port=2
  TireComp : Outport  Orientation=left  Port=3
  wires:
  " (36)"/1 -> Fcn/1  "Strut_force"
  " (99)"/1 -> " (36)"/1  "Delta_force"
  Stiffness vs Deflection/1 -> " (99)"/2  "Stiffness"
  Fcn/1 -> S2dot/1
  S/1 -> " (99)1"/2, Stiffness vs Deflection/1
  " (96)1"/1 -> " (99)"/1, TireForce/1  "TireForce"
  " (99)1"/1 -> Saturation/1  "TireComp"
  Hagl/1 -> " (99)1"/1
  Saturation/1 -> " (96)1"/1, TireComp/1
  Product/1 -> " (96)"/1
  Abs/1 -> Product/2
  Sdot/1 -> Product/1, Abs/1, " (96)2"/1
  " (96)"/1 -> " (99)2"/1  "Damping"
  " (96)2"/1 -> " (99)2"/2
  " (99)2"/1 -> " (36)"/2

== system AeroLib/GroundReactions/Landing_Gear/Nose Gear Dynamics/LGEAR States ==
  S2dot : Inport  Port=1  PortDimensions=1  SampleTime=[Flight_TimeStep,0]  LatchInput=off
  NG_S : Integrator  LimitOutput=on  UpperSaturationLimit=Strut_Limit  LowerSaturationLimit=0
  NG_Sdot : Integrator  UpperSaturationLimit=100  LowerSaturationLimit=-100
  Sdot : Outport
  S : Outport  Port=2
  wires:
  NG_Sdot/1 -> Sdot/1, NG_S/1  "Sdot"
  S2dot/1 -> NG_Sdot/1
  NG_S/1 -> S/1  "S"

== system AeroLib/GroundReactions/Landing_Gear/Nose Gear Dynamics/NoseWheelAngle ==
  Vtg : Inport  Port=1  LatchInput=off
  Caster : Inport  Port=2  LatchInput=off
  NoseWheelAng : Inport  Port=3  LatchInput=off
  Fcn : Fcn  Expr=atan2(u(2),u(1))*180/pi
  Switch : Switch
  Out1 : Outport
  wires:
  Fcn/1 -> Switch/1
  Vtg/1 -> Fcn/1
  Caster/1 -> Switch/2
  Switch/1 -> Out1/1
  NoseWheelAng/1 -> Switch/3

== system AeroLib/GroundReactions/Landing_Gear/Right Main Gear Dynamics/Ground_Tire Contact ==
  DCbg : Inport  Port=1  LatchInput=off
  VelB : Inport  Port=2  LatchInput=off
  RatesB : Inport  Port=3  LatchInput=off
  Sdot : Inport  Port=4  LatchInput=off
  S : Inport  Port=5  LatchInput=off
  TireComp : Inport  Port=6  LatchInput=off
  Conf_Tire_RposRmg : Inport  Port=7  LatchInput=off
  " (97)1" : Sum  Inputs=|+-  SaturateOnIntegerOverflow=on  InputSameDT=on
  " (97)2" : Sum  Inputs=|++  SaturateOnIntegerOverflow=on  InputSameDT=on
  " (98) Mux_3" : Mux  Inputs=3
  3x3 cross product : aerospace/Axes Transformations/3x3 cross product
  Fcn : Fcn  Expr=u(1)
  Fcn1 : Fcn  Expr=u(2)
  Fcn2 : Fcn  Expr=u(3)-u(4)-u(5)
  Product1 : Product  Multiplication=Matrix(*)  SaturateOnIntegerOverflow=on  InputSameDT=on
  Tire Position Body_Axis (95) Mux_1 : Mux  Inputs=3
  Tire Transl_Speed Body_Axis (96) Demux1 : Demux  Outputs=3
  Tire Transl_Speed Body_Axis (96) Mux_2 : Mux  Inputs=3
  Rtb : Outport
  Vtg : Outport  Port=2
  wires:
  Tire Transl_Speed Body_Axis (96) Demux1/1 -> Tire Transl_Speed Body_Axis (96) Mux_2/1
  Tire Transl_Speed Body_Axis (96) Demux1/2 -> Tire Transl_Speed Body_Axis (96) Mux_2/2
  Tire Transl_Speed Body_Axis (96) Demux1/3 -> " (97)1"/1
  Sdot/1 -> " (97)1"/2  "Sdot"
  " (97)1"/1 -> Tire Transl_Speed Body_Axis (96) Mux_2/3
  Tire Transl_Speed Body_Axis (96) Mux_2/1 -> " (97)2"/1  "Vtbtrans"
  TireComp/1 -> Tire Position Body_Axis (95) Mux_1/3
  S/1 -> Tire Position Body_Axis (95) Mux_1/2
  Tire Position Body_Axis (95) Mux_1/1 -> Fcn/1, Fcn1/1, Fcn2/1
  Fcn/1 -> " (98) Mux_3"/1
  Fcn1/1 -> " (98) Mux_3"/2
  Fcn2/1 -> " (98) Mux_3"/3
  " (98) Mux_3"/1 -> Rtb/1, 3x3 cross product/1  "Rtb"
  3x3 cross product/1 -> " (97)2"/2
  " (97)2"/1 -> Product1/2  "Vtb"
  DCbg/1 -> Product1/1
  Product1/1 -> Vtg/1
  Conf_Tire_RposRmg/1 -> Tire Position Body_Axis (95) Mux_1/1
  VelB/1 -> Tire Transl_Speed Body_Axis (96) Demux1/1
  RatesB/1 -> 3x3 cross product/2

== system AeroLib/GroundReactions/Landing_Gear/Right Main Gear Dynamics/Ground_Tire Friction ==
  TireForce : Inport  Port=1  PortDimensions=1  LatchInput=off
  Vtg : Inport  Port=2  PortDimensions=3  LatchInput=off
  Brake : Inport  Port=3  PortDimensions=1  LatchInput=off
  Demux : Demux  Outputs=3
  Friction Coeff : Subsystem
  Terminator : Terminator
  MUside : Outport
  MUeff : Outport  Port=2
  wires:
  Friction Coeff/1(MUside) -> MUside/1
  Friction Coeff/2(MUeff) -> MUeff/1
  Brake/1 -> Friction Coeff/1(Brake)
  Vtg/1 -> Demux/1
  TireForce/1 -> Friction Coeff/4(TireForce)
  Demux/1 -> Friction Coeff/2(Ug)  "Ug"
  Demux/2 -> Friction Coeff/3(Vg)  "Vg"
  Demux/3 -> Terminator/1  "Wg"

== system AeroLib/GroundReactions/Landing_Gear/Right Main Gear Dynamics/LGEAR Accelerations ==
  Hagl : Inport  Orientation=left  Port=1  LatchInput=off
  Sdot : Inport  Orientation=left  Port=2  PortDimensions=1  LatchInput=off
  S : Inport  Orientation=left  Port=3  PortDimensions=1  LatchInput=off
  " (36)" : Sum  Orientation=left  Inputs=+-  SaturateOnIntegerOverflow=on  InputSameDT=on
  " (96)" : Gain  Orientation=left  Gain=Damping  SaturateOnIntegerOverflow=on
  " (96)1" : Gain  Orientation=left  Gain=Tire_Stiffness  SaturateOnIntegerOverflow=on
  " (96)2" : Gain  Orientation=left  Gain=CFriction  SaturateOnIntegerOverflow=on
  " (99)" : Sum  Orientation=left  Inputs=+-  SaturateOnIntegerOverflow=on  InputSameDT=on
  " (99)1" : Sum  Orientation=left  Inputs=|+-  SaturateOnIntegerOverflow=on  InputSameDT=on
  " (99)2" : Sum  Orientation=left  SaturateOnIntegerOverflow=on  InputSameDT=on
  Abs : Abs  Orientation=left  SaturateOnIntegerOverflow=on
  Fcn : Fcn  Orientation=left  Expr=u/Mass/AccFactor
  Product : Product  Orientation=left  SaturateOnIntegerOverflow=on  InputSameDT=on
  Saturation : Saturate  Orientation=left  UpperLimit=TireMaxComp  LowerLimit=0
  Stiffness vs Deflection : Lookup  Orientation=left  DialogController=Simulink.DDGSource  InputValues=Strut_Deflection  OutputValues=Strut_Stiffness  SaturateOnIntegerOverflow=on
  TireForce : Outport  Orientation=left
  S2dot : Outport  Orientation=left  Port=2
  TireComp : Outport  Orientation=left  Port=3
  wires:
  " (36)"/1 -> Fcn/1  "Strut_force"
  " (99)"/1 -> " (36)"/1  "Delta_force"
  Stiffness vs Deflection/1 -> " (99)"/2  "Stiffness"
  Fcn/1 -> S2dot/1
  S/1 -> " (99)1"/2, Stiffness vs Deflection/1
  " (96)1"/1 -> " (99)"/1, TireForce/1  "TireForce"
  " (99)1"/1 -> Saturation/1  "TireComp"
  Hagl/1 -> " (99)1"/1
  Saturation/1 -> " (96)1"/1, TireComp/1
  Product/1 -> " (96)"/1
  Abs/1 -> Product/2
  Sdot/1 -> Product/1, Abs/1, " (96)2"/1
  " (96)"/1 -> " (99)2"/1  "Damping"
  " (96)2"/1 -> " (99)2"/2
  " (99)2"/1 -> " (36)"/2

== system AeroLib/GroundReactions/Landing_Gear/Right Main Gear Dynamics/LGEAR States ==
  S2dot : Inport  Port=1  PortDimensions=1  SampleTime=[Flight_TimeStep,0]  LatchInput=off
  RMG_S : Integrator  LimitOutput=on  UpperSaturationLimit=Strut_Limit  LowerSaturationLimit=0
  RMG_Sdot : Integrator  UpperSaturationLimit=100  LowerSaturationLimit=-100
  Sdot : Outport
  S : Outport  Port=2
  wires:
  RMG_S/1 -> S/1  "S"
  S2dot/1 -> RMG_Sdot/1
  RMG_Sdot/1 -> RMG_S/1, Sdot/1  "Sdot"

== system AeroLib/Propulsion/Piston_Engine_Propeller/Power_Limit/Rpm_Limit ==
  deltaPower : Inport  Port=1  LatchInput=off
  Rpm : Inport  Port=2  LatchInput=off
  Fcn5 : Fcn  Expr=u(1) > 0 && u(2) > Eng.LimRpm
  Fcn6 : Fcn  Expr=(Eng.LimRpm-u(2))/5
  Mux2 : Mux  Inputs=2
  Product2 : Product  SaturateOnIntegerOverflow=on  InputSameDT=on
  Rpm_Command : Outport
  wires:
  Product2/1 -> Rpm_Command/1
  Rpm/1 -> Mux2/2
  deltaPower/1 -> Mux2/1
  Mux2/1 -> Fcn6/1, Fcn5/1
  Fcn5/1 -> Product2/1
  Fcn6/1 -> Product2/2

== system AeroLib/Sensors/Inertial_Reference_Unit/Accelerometers/Sensors ==
  Xdist : Inport  Port=1  LatchInput=off
  Ydist : Inport  Port=2  LatchInput=off
  Latitude : Inport  Port=3  LatchInput=off
  Longitude : Inport  Port=4  LatchInput=off
  From_Reset : Inport  Port=5  LatchInput=off
  SensorsOFF : Subsystem
  Simple_Sensor : AeroLib/Sensors/Simple_Sensor  Var=Sensors.IRU.Acc.XYdist.Var  Seed=Sensors.IRU.Acc.XYdist.Seed  Max=inf  Min=-inf  Time_Const=Sensors.IRU.Acc.XYdist.TimeConst
  Simple_Sensor1 : AeroLib/Sensors/Simple_Sensor  Var=Sensors.IRU.Acc.XYdist.Var  Seed=Sensors.IRU.Acc.XYdist.Seed  Max=inf  Min=-inf  Time_Const=Sensors.IRU.Acc.XYdist.TimeConst
  Simple_Sensor2 : AeroLib/Sensors/Simple_Sensor  Var=Sensors.IRU.Acc.LatLon.Var  Seed=Sensors.IRU.Acc.LatLon.Seed  Max=90  Min=-90  Time_Const=Sensors.IRU.Acc.LatLon.TimeConst
  Simple_Sensor3 : AeroLib/Sensors/Simple_Sensor  Var=Sensors.IRU.Acc.LatLon.Var  Seed=Sensors.IRU.Acc.LatLon.Seed  Max=180  Min=-180  Time_Const=Sensors.IRU.Acc.LatLon.TimeConst
  Switch{,1..3} (4 alike) : Switch  Threshold=0.5  SaturateOnIntegerOverflow=on  InputSameDT=on
  X : Outport
  Y : Outport  Port=2
  Lat : Outport  Port=3
  Lon : Outport  Port=4
  wires:
  SensorsOFF/1(SensorsOFF) -> Switch/2, Switch1/2, Switch2/2, Switch3/2
  From_Reset/1 -> Simple_Sensor2/3, Simple_Sensor3/3, Simple_Sensor1/3, Simple_Sensor/3
  Simple_Sensor/1 -> Switch/3
  Simple_Sensor1/1 -> Switch1/3
  Simple_Sensor2/1 -> Switch2/3
  Simple_Sensor3/1 -> Switch3/3
  Switch3/1 -> Lon/1
  Longitude/1 -> Simple_Sensor3/2, Switch3/1, Simple_Sensor3/1
  Switch2/1 -> Lat/1
  Latitude/1 -> Simple_Sensor2/2, Switch2/1, Simple_Sensor2/1
  Switch1/1 -> Y/1
  Ydist/1 -> Switch1/1, Simple_Sensor1/1, Simple_Sensor1/2
  Switch/1 -> X/1
  Xdist/1 -> Simple_Sensor/2, Switch/1, Simple_Sensor/1

== system AeroLib/Sensors/Inertial_Reference_Unit/Airspeed_Detectors/SensorsOFF ==
  Clock : Clock
      settings: Decimation=10
  Constant1 : Constant  Value=Flight_SensorsON
  Fcn : Fcn  Expr=u <= 0+eps
  or : Logic  Operator=OR
  or1 : Logic  Operator=NOT
  SensorsOFF : Outport
  wires:
  or1/1 -> or/1
  or/1 -> SensorsOFF/1
  Fcn/1 -> or/2
  Constant1/1 -> or1/1  "DT"
  Clock/1 -> Fcn/1

== system AeroLib/Sensors/Inertial_Reference_Unit/Altitude_Sensors/SensorsOFF ==
  Clock : Clock
      settings: Decimation=10
  Constant1 : Constant  Value=Flight_SensorsON
  Fcn : Fcn  Expr=u <= 0+eps
  or : Logic  Operator=OR
  or1 : Logic  Operator=NOT
  SensorsOFF : Outport
  wires:
  or1/1 -> or/1
  or/1 -> SensorsOFF/1
  Fcn/1 -> or/2
  Constant1/1 -> or1/1  "DT"
  Clock/1 -> Fcn/1

== system AeroLib/Sensors/Inertial_Reference_Unit/Flow_Incidence_Angle_Sensors/SensorsOFF ==
  Clock : Clock
      settings: Decimation=10
  Constant1 : Constant  Value=Flight_SensorsON
  Fcn : Fcn  Expr=u <= 0+eps
  or : Logic  Operator=OR
  or1 : Logic  Operator=NOT
  SensorsOFF : Outport
  wires:
  or1/1 -> or/1
  or/1 -> SensorsOFF/1
  Fcn/1 -> or/2
  Constant1/1 -> or1/1  "DT"
  Clock/1 -> Fcn/1

== system AeroLib/Aerodynamics/Aerodynamics_Pioneer/Aero_Dynamic_Coefficients/Aero LatDyn_Coef/DynCoef Roll_Rate (4) ==
  p_hat : Inport  Port=1  LatchInput=off
  Constant : Constant  Value=Aero.CY.Prate
  Constant1 : Constant  Value=Aero.CR.Prate
  Constant2 : Constant  Value=Aero.CN.Prate
  Demux : Demux  Outputs=3
  Mux : Mux  Inputs=3
  Product1 : Product  SaturateOnIntegerOverflow=on  InputSameDT=on
  CYp : Outport
  CRp : Outport  Port=2
  CNp : Outport  Port=3
  wires:
  Demux/1 -> CYp/1
  Demux/2 -> CRp/1
  Demux/3 -> CNp/1
  Product1/1 -> Demux/1
  p_hat/1 -> Product1/2
  Mux/1 -> Product1/1
  Constant2/1 -> Mux/3
  Constant1/1 -> Mux/2
  Constant/1 -> Mux/1

== system AeroLib/Aerodynamics/Aerodynamics_Pioneer/Aero_Dynamic_Coefficients/Aero LatDyn_Coef/DynCoef Yaw_Rate ==
  r_hat : Inport  Port=1  LatchInput=off
  Constant : Constant  Value=Aero.CY.Rrate
  Constant1 : Constant  Value=Aero.CR.Rrate
  Constant2 : Constant  Value=Aero.CN.Rrate
  Demux : Demux  Outputs=3
  Mux : Mux  Inputs=3
  Product1 : Product  SaturateOnIntegerOverflow=on  InputSameDT=on
  CYr : Outport
  CRr : Outport  Port=2
  CNr : Outport  Port=3
  wires:
  Demux/1 -> CYr/1
  Demux/2 -> CRr/1
  Demux/3 -> CNr/1
  Product1/1 -> Demux/1
  r_hat/1 -> Product1/2
  Mux/1 -> Product1/1
  Constant2/1 -> Mux/3
  Constant1/1 -> Mux/2
  Constant/1 -> Mux/1
